simulink model "augumented_slx"  (R2023a)
settings: Solver=VariableStepAuto  StartTime=0.0  StopTime=10.0  RelTol=1e-3
values from neighbouring files (symbols this model uses):
  G_den = cell2mat(G_den)    [augmented.m]
  G_num = cell2mat(G_num)    [augmented.m]
  K_den = cell2mat(K_den)    [augmented.m]
  K_num = cell2mat(K_num)    [augmented.m]
settings Model: Creator=enric  LastModifiedBy=enric

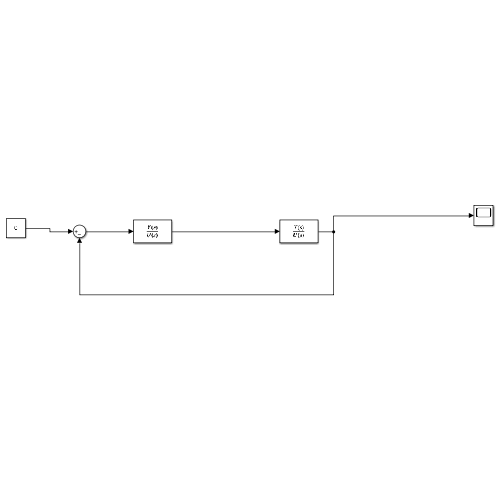
[thumbnail: Simulink's stored preview of the top-level diagram]
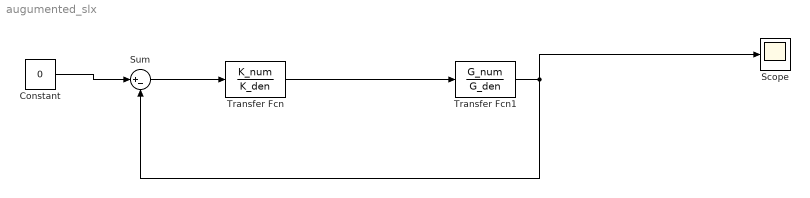
== system augumented_slx ==
  Constant : Constant  Value=0
  Scope : Scope
  Sum : Sum  Inputs=|+-
  Transfer Fcn : TransferFcn  Numerator=K_num  Denominator=K_den
  Transfer Fcn1 : TransferFcn  Numerator=G_num  Denominator=G_den
  wires:
  Transfer Fcn/1 -> Transfer Fcn1/1
  Sum/1 -> Transfer Fcn/1
  Constant/1 -> Sum/1
  Transfer Fcn1/1 -> Scope/1, Sum/2
